simulink model "W02_Base_Map_PB_cs"  (R2019a)
settings: Solver=FixedStepDiscrete  StartTime=0.0  StopTime=inf  FixedStep=1/300  RelTol=1e-3
PreLoadFcn:
  | mbxruntime.callbacks.PreLoadFcn(bdroot);
  | check_NUTS_defined
  | model_closed = 0;
  | assignin('base',['model_closed_' bdroot],false);
PostLoadFcn:
  | mbxruntime.callbacks.PostLoadFcn(bdroot);
InitFcn:
  | mbxruntime.callbacks.InitFcn(bdroot);
StartFcn:
  | mbxruntime.callbacks.StartFcn(bdroot);
StopFcn:
  | mbxruntime.callbacks.StopFcn(bdroot);;
  | 
model workspace: external: MAT-File .\W02_Base_Map_PB_cs_hws.mat (data not in the file)
undefined symbols (not defined in the file or in its folder): DiscIntNeverNeededParam, Header, InitImageOutputDir, mbxruntime, Orientation, Pose, Poses, Poses_SL_Info, Position, tabledata
libraries: PBCSimulinkLibrary x57, simulink_extras x9, PreScanSimulinkLibrary x6, robotlib x6, PreScanUsefulBlocks x4, sharedtransform x3, aerolibutil x2, visionconversions x1, visionsinks x1
(part 3 of 7)

== system W02_Base_Map_PB_cs/TrafficLightRoadSideNL_1 ==
  note: Light SPD Resources
      |
      |  0: CIE_A_standard_incandescent_illuminant.txt
      |  1: CIE_A_standard_incandescent_illuminant.txt_x_R255_G191_B000.txt
      |  2: CIE_A_standard_incandescent_illuminant.txt_x_R583_G047_B000.txt
      |  3: CIE_F12_standard_fluorescent_illuminant.txt
      |  4: Illuminant_D65.txt
      |  5: Light_SPD_H1_12_8V_Filament.txt
      |  6: Light_SPD_H1_13_2V_Filament.txt
      |  7: Light_SPD_H11_12V_Filament.txt
      |  8: Light_SPD_H7_12_8V_Filament.txt
      |  9: Light_SPD_H7_13_2V_Filament.txt
      | 10: Light_SPD_H8_13_2V_Filament.txt
      | 11: Light_SPD_Halogen.txt
      | 12: Light_SPD_High_Power_LED.txt
      | 13: Light_SPD_HPS_High_Pressure_Sodium.txt
      | 14: Light_SPD_incandescent_traffic_signal_amber.txt
      | 15: Light_SPD_incandescent_traffic_signal_green.txt
      | 16: Light_SPD_incandescent_traffic_signal_red.txt
      | 17: Light_SPD_LED_D1S_HID.txt
      | 18: Light_SPD_LED_traffic_signal_amber.txt
      | 19: Light_SPD_LED_traffic_signal_green.txt
      | 20: Light_SPD_LED_traffic_signal_red.txt
      | 21: Light_SPD_LPS_Low_Pressure_Sodium.txt
      | 22: Light_SPD_Mercury.txt
      | 23: Light_SPD_Reddish_Neon_Sign.txt
      | 24: Noma_Twister_Blue_13W_120V.txt
      | 25: Philips_Blue_Golite_P1_Apollo_1750Lux.txt
      | 26: SPD_flat_1.0.txt
  note: Light SPD Resources
  Ground_1 : Ground
  Ground_2 : Ground
  Ground_3 : Ground
  TrafficLightRoadSideNL_1_Casing.LightGreen_Control_Mux : Subsystem  Tag=mux/plugin/LightSignals
  TrafficLightRoadSideNL_1_Casing.LightGreen_Power : Constant  Tag=TrafficLightRoadSideNL_1_Casing.LightGreen_Power  Value=0
  TrafficLightRoadSideNL_1_Casing.LightGreen_SPDIndex : Constant  Tag=TrafficLightRoadSideNL_1_Casing.LightGreen_SPDIndex  Value=15
  TrafficLightRoadSideNL_1_Casing.LightOrange_Control_Mux : Subsystem  Tag=mux/plugin/LightSignals
  TrafficLightRoadSideNL_1_Casing.LightOrange_Power : Constant  Tag=TrafficLightRoadSideNL_1_Casing.LightOrange_Power  Value=0
  TrafficLightRoadSideNL_1_Casing.LightOrange_SPDIndex : Constant  Tag=TrafficLightRoadSideNL_1_Casing.LightOrange_SPDIndex  Value=14
  TrafficLightRoadSideNL_1_Casing.LightRed_Control_Mux : Subsystem  Tag=mux/plugin/LightSignals
  TrafficLightRoadSideNL_1_Casing.LightRed_Power : Constant  Tag=TrafficLightRoadSideNL_1_Casing.LightRed_Power  Value=0
  TrafficLightRoadSideNL_1_Casing.LightRed_SPDIndex : Constant  Tag=TrafficLightRoadSideNL_1_Casing.LightRed_SPDIndex  Value=16
  VISUCasingLights_Mux : Subsystem  Tag=mux/VisuCasingLights  mask(PreScan User Interface: VisuTrafficLight){}
      mask help:
      | The VisuTrafficLight block provides a way to animate traffic lights: switch on and off individual lights.
      |
      | For more information, please click Help.
      mask Help: eval('openHelp(731)')
  VISUCasingLights_TrafficLightRoadSideNL_1 : Outport  Tag=outport/VisuCasingLights  SampleTime=1/300
  TrafficLightRoadSideNL_1_Casing.LightRed_Control : Outport  Tag=outport/plugin/sfun_PBCLight  Port=2  OutDataTypeStr=Bus: PRESCAN_PBCLIGHT_DATA  PortDimensions=1  SampleTime=0.05
  TrafficLightRoadSideNL_1_Casing.LightOrange_Control : Outport  Tag=outport/plugin/sfun_PBCLight  Port=3  OutDataTypeStr=Bus: PRESCAN_PBCLIGHT_DATA  PortDimensions=1  SampleTime=0.05
  TrafficLightRoadSideNL_1_Casing.LightGreen_Control : Outport  Tag=outport/plugin/sfun_PBCLight  Port=4  OutDataTypeStr=Bus: PRESCAN_PBCLIGHT_DATA  PortDimensions=1  SampleTime=0.05
  wires:
  VISUCasingLights_Mux/1(VISUCasingLights_TrafficLightRoadSideNL_1) -> VISUCasingLights_TrafficLightRoadSideNL_1/1
  TrafficLightRoadSideNL_1_Casing.LightRed_Control_Mux/1(Bus) -> TrafficLightRoadSideNL_1_Casing.LightRed_Control/1
  TrafficLightRoadSideNL_1_Casing.LightRed_SPDIndex/1 -> TrafficLightRoadSideNL_1_Casing.LightRed_Control_Mux/1(SPDIndex [-])
  TrafficLightRoadSideNL_1_Casing.LightRed_Power/1 -> TrafficLightRoadSideNL_1_Casing.LightRed_Control_Mux/2(Power [W])
  TrafficLightRoadSideNL_1_Casing.LightOrange_Control_Mux/1(Bus) -> TrafficLightRoadSideNL_1_Casing.LightOrange_Control/1
  TrafficLightRoadSideNL_1_Casing.LightOrange_SPDIndex/1 -> TrafficLightRoadSideNL_1_Casing.LightOrange_Control_Mux/1(SPDIndex [-])
  TrafficLightRoadSideNL_1_Casing.LightOrange_Power/1 -> TrafficLightRoadSideNL_1_Casing.LightOrange_Control_Mux/2(Power [W])
  TrafficLightRoadSideNL_1_Casing.LightGreen_Control_Mux/1(Bus) -> TrafficLightRoadSideNL_1_Casing.LightGreen_Control/1
  TrafficLightRoadSideNL_1_Casing.LightGreen_SPDIndex/1 -> TrafficLightRoadSideNL_1_Casing.LightGreen_Control_Mux/1(SPDIndex [-])
  TrafficLightRoadSideNL_1_Casing.LightGreen_Power/1 -> TrafficLightRoadSideNL_1_Casing.LightGreen_Control_Mux/2(Power [W])
  Ground_1/1 -> VISUCasingLights_Mux/1(Green [-])
  Ground_2/1 -> VISUCasingLights_Mux/2(Orange [-])
  Ground_3/1 -> VISUCasingLights_Mux/3(Red [-])

== system W02_Base_Map_PB_cs/TrafficLightRoadSideNL_1_Casing.LightGreen_Control ==
  TrafficLightRoadSideNL_1_Casing.LightGreen_Control : Inport  Tag=inport/plugin/sfun_PBCLight  OutDataTypeStr=Bus: PRESCAN_PBCLIGHT_DATA  PortDimensions=1  SampleTime=0.05  BusOutputAsStruct=on
  Actuator : S-Function  LoadFcn=addpath 'C:/Program Files/Simcenter Prescan/Prescan_2019.2/Plugins/PBCameraPlugin/matlab';addpath 'C:/Program Files/Simcenter Prescan/Prescan_2019.2/Plugins/PBCameraPlugin/bin';load('PreScanPBCLightData.mat');  FunctionName=sfun_PBCLight  Parameters=lightID, timestepMask  SFunctionDeploymentMode=off  EnableBusSupport=off  mask(Physics Based Camera plugin block){lightID=2, timestepMask=0.05}
      mask prompts: lightID "Light ID:"; timestepMask "MATLAB timestep:"
      mask help: Light Control I/O
      mask Help: eval('openHelp(6500)')
      mask Display: image(imread('ico_PBCControl.png'))
  wires:
  TrafficLightRoadSideNL_1_Casing.LightGreen_Control/1 -> Actuator/1

== system W02_Base_Map_PB_cs/TrafficLightRoadSideNL_1_Casing.LightOrange_Control ==
  TrafficLightRoadSideNL_1_Casing.LightOrange_Control : Inport  Tag=inport/plugin/sfun_PBCLight  OutDataTypeStr=Bus: PRESCAN_PBCLIGHT_DATA  PortDimensions=1  SampleTime=0.05  BusOutputAsStruct=on
  Actuator : S-Function  LoadFcn=addpath 'C:/Program Files/Simcenter Prescan/Prescan_2019.2/Plugins/PBCameraPlugin/matlab';addpath 'C:/Program Files/Simcenter Prescan/Prescan_2019.2/Plugins/PBCameraPlugin/bin';load('PreScanPBCLightData.mat');  FunctionName=sfun_PBCLight  Parameters=lightID, timestepMask  SFunctionDeploymentMode=off  EnableBusSupport=off  mask(Physics Based Camera plugin block){lightID=1, timestepMask=0.05}
      mask prompts: lightID "Light ID:"; timestepMask "MATLAB timestep:"
      mask help: Light Control I/O
      mask Help: eval('openHelp(6500)')
      mask Display: image(imread('ico_PBCControl.png'))
  wires:
  TrafficLightRoadSideNL_1_Casing.LightOrange_Control/1 -> Actuator/1

== system W02_Base_Map_PB_cs/TrafficLightRoadSideNL_1_Casing.LightRed_Control ==
  TrafficLightRoadSideNL_1_Casing.LightRed_Control : Inport  Tag=inport/plugin/sfun_PBCLight  OutDataTypeStr=Bus: PRESCAN_PBCLIGHT_DATA  PortDimensions=1  SampleTime=0.05  BusOutputAsStruct=on
  Actuator : S-Function  LoadFcn=addpath 'C:/Program Files/Simcenter Prescan/Prescan_2019.2/Plugins/PBCameraPlugin/matlab';addpath 'C:/Program Files/Simcenter Prescan/Prescan_2019.2/Plugins/PBCameraPlugin/bin';load('PreScanPBCLightData.mat');  FunctionName=sfun_PBCLight  Parameters=lightID, timestepMask  SFunctionDeploymentMode=off  EnableBusSupport=off  mask(Physics Based Camera plugin block){lightID=0, timestepMask=0.05}
      mask prompts: lightID "Light ID:"; timestepMask "MATLAB timestep:"
      mask help: Light Control I/O
      mask Help: eval('openHelp(6500)')
      mask Display: image(imread('ico_PBCControl.png'))
  wires:
  TrafficLightRoadSideNL_1_Casing.LightRed_Control/1 -> Actuator/1

== system W02_Base_Map_PB_cs/TrafficLightRoadSideNL_2 ==
  note: Light SPD Resources
      |
      |  0: CIE_A_standard_incandescent_illuminant.txt
      |  1: CIE_A_standard_incandescent_illuminant.txt_x_R255_G191_B000.txt
      |  2: CIE_A_standard_incandescent_illuminant.txt_x_R583_G047_B000.txt
      |  3: CIE_F12_standard_fluorescent_illuminant.txt
      |  4: Illuminant_D65.txt
      |  5: Light_SPD_H1_12_8V_Filament.txt
      |  6: Light_SPD_H1_13_2V_Filament.txt
      |  7: Light_SPD_H11_12V_Filament.txt
      |  8: Light_SPD_H7_12_8V_Filament.txt
      |  9: Light_SPD_H7_13_2V_Filament.txt
      | 10: Light_SPD_H8_13_2V_Filament.txt
      | 11: Light_SPD_Halogen.txt
      | 12: Light_SPD_High_Power_LED.txt
      | 13: Light_SPD_HPS_High_Pressure_Sodium.txt
      | 14: Light_SPD_incandescent_traffic_signal_amber.txt
      | 15: Light_SPD_incandescent_traffic_signal_green.txt
      | 16: Light_SPD_incandescent_traffic_signal_red.txt
      | 17: Light_SPD_LED_D1S_HID.txt
      | 18: Light_SPD_LED_traffic_signal_amber.txt
      | 19: Light_SPD_LED_traffic_signal_green.txt
      | 20: Light_SPD_LED_traffic_signal_red.txt
      | 21: Light_SPD_LPS_Low_Pressure_Sodium.txt
      | 22: Light_SPD_Mercury.txt
      | 23: Light_SPD_Reddish_Neon_Sign.txt
      | 24: Noma_Twister_Blue_13W_120V.txt
      | 25: Philips_Blue_Golite_P1_Apollo_1750Lux.txt
      | 26: SPD_flat_1.0.txt
  note: Light SPD Resources
  Ground_1 : Ground
  Ground_2 : Ground
  Ground_3 : Ground
  TrafficLightRoadSideNL_2_Casing.LightGreen_Control_Mux : Subsystem  Tag=mux/plugin/LightSignals
  TrafficLightRoadSideNL_2_Casing.LightGreen_Power : Constant  Tag=TrafficLightRoadSideNL_2_Casing.LightGreen_Power  Value=0
  TrafficLightRoadSideNL_2_Casing.LightGreen_SPDIndex : Constant  Tag=TrafficLightRoadSideNL_2_Casing.LightGreen_SPDIndex  Value=15
  TrafficLightRoadSideNL_2_Casing.LightOrange_Control_Mux : Subsystem  Tag=mux/plugin/LightSignals
  TrafficLightRoadSideNL_2_Casing.LightOrange_Power : Constant  Tag=TrafficLightRoadSideNL_2_Casing.LightOrange_Power  Value=0
  TrafficLightRoadSideNL_2_Casing.LightOrange_SPDIndex : Constant  Tag=TrafficLightRoadSideNL_2_Casing.LightOrange_SPDIndex  Value=14
  TrafficLightRoadSideNL_2_Casing.LightRed_Control_Mux : Subsystem  Tag=mux/plugin/LightSignals
  TrafficLightRoadSideNL_2_Casing.LightRed_Power : Constant  Tag=TrafficLightRoadSideNL_2_Casing.LightRed_Power  Value=0
  TrafficLightRoadSideNL_2_Casing.LightRed_SPDIndex : Constant  Tag=TrafficLightRoadSideNL_2_Casing.LightRed_SPDIndex  Value=16
  VISUCasingLights_Mux : Subsystem  Tag=mux/VisuCasingLights  mask(PreScan User Interface: VisuTrafficLight){}
      mask help:
      | The VisuTrafficLight block provides a way to animate traffic lights: switch on and off individual lights.
      |
      | For more information, please click Help.
      mask Help: eval('openHelp(731)')
  VISUCasingLights_TrafficLightRoadSideNL_2 : Outport  Tag=outport/VisuCasingLights  SampleTime=1/300
  TrafficLightRoadSideNL_2_Casing.LightRed_Control : Outport  Tag=outport/plugin/sfun_PBCLight  Port=2  OutDataTypeStr=Bus: PRESCAN_PBCLIGHT_DATA  PortDimensions=1  SampleTime=0.05
  TrafficLightRoadSideNL_2_Casing.LightOrange_Control : Outport  Tag=outport/plugin/sfun_PBCLight  Port=3  OutDataTypeStr=Bus: PRESCAN_PBCLIGHT_DATA  PortDimensions=1  SampleTime=0.05
  TrafficLightRoadSideNL_2_Casing.LightGreen_Control : Outport  Tag=outport/plugin/sfun_PBCLight  Port=4  OutDataTypeStr=Bus: PRESCAN_PBCLIGHT_DATA  PortDimensions=1  SampleTime=0.05
  wires:
  VISUCasingLights_Mux/1(VISUCasingLights_TrafficLightRoadSideNL_2) -> VISUCasingLights_TrafficLightRoadSideNL_2/1
  TrafficLightRoadSideNL_2_Casing.LightRed_Control_Mux/1(Bus) -> TrafficLightRoadSideNL_2_Casing.LightRed_Control/1
  TrafficLightRoadSideNL_2_Casing.LightRed_SPDIndex/1 -> TrafficLightRoadSideNL_2_Casing.LightRed_Control_Mux/1(SPDIndex [-])
  TrafficLightRoadSideNL_2_Casing.LightRed_Power/1 -> TrafficLightRoadSideNL_2_Casing.LightRed_Control_Mux/2(Power [W])
  TrafficLightRoadSideNL_2_Casing.LightOrange_Control_Mux/1(Bus) -> TrafficLightRoadSideNL_2_Casing.LightOrange_Control/1
  TrafficLightRoadSideNL_2_Casing.LightOrange_SPDIndex/1 -> TrafficLightRoadSideNL_2_Casing.LightOrange_Control_Mux/1(SPDIndex [-])
  TrafficLightRoadSideNL_2_Casing.LightOrange_Power/1 -> TrafficLightRoadSideNL_2_Casing.LightOrange_Control_Mux/2(Power [W])
  TrafficLightRoadSideNL_2_Casing.LightGreen_Control_Mux/1(Bus) -> TrafficLightRoadSideNL_2_Casing.LightGreen_Control/1
  TrafficLightRoadSideNL_2_Casing.LightGreen_SPDIndex/1 -> TrafficLightRoadSideNL_2_Casing.LightGreen_Control_Mux/1(SPDIndex [-])
  TrafficLightRoadSideNL_2_Casing.LightGreen_Power/1 -> TrafficLightRoadSideNL_2_Casing.LightGreen_Control_Mux/2(Power [W])
  Ground_1/1 -> VISUCasingLights_Mux/1(Green [-])
  Ground_2/1 -> VISUCasingLights_Mux/2(Orange [-])
  Ground_3/1 -> VISUCasingLights_Mux/3(Red [-])

== system W02_Base_Map_PB_cs/TrafficLightRoadSideNL_2_Casing.LightGreen_Control ==
  TrafficLightRoadSideNL_2_Casing.LightGreen_Control : Inport  Tag=inport/plugin/sfun_PBCLight  OutDataTypeStr=Bus: PRESCAN_PBCLIGHT_DATA  PortDimensions=1  SampleTime=0.05  BusOutputAsStruct=on
  Actuator : S-Function  LoadFcn=addpath 'C:/Program Files/Simcenter Prescan/Prescan_2019.2/Plugins/PBCameraPlugin/matlab';addpath 'C:/Program Files/Simcenter Prescan/Prescan_2019.2/Plugins/PBCameraPlugin/bin';load('PreScanPBCLightData.mat');  FunctionName=sfun_PBCLight  Parameters=lightID, timestepMask  SFunctionDeploymentMode=off  EnableBusSupport=off  mask(Physics Based Camera plugin block){lightID=5, timestepMask=0.05}
      mask prompts: lightID "Light ID:"; timestepMask "MATLAB timestep:"
      mask help: Light Control I/O
      mask Help: eval('openHelp(6500)')
      mask Display: image(imread('ico_PBCControl.png'))
  wires:
  TrafficLightRoadSideNL_2_Casing.LightGreen_Control/1 -> Actuator/1

== system W02_Base_Map_PB_cs/TrafficLightRoadSideNL_2_Casing.LightOrange_Control ==
  TrafficLightRoadSideNL_2_Casing.LightOrange_Control : Inport  Tag=inport/plugin/sfun_PBCLight  OutDataTypeStr=Bus: PRESCAN_PBCLIGHT_DATA  PortDimensions=1  SampleTime=0.05  BusOutputAsStruct=on
  Actuator : S-Function  LoadFcn=addpath 'C:/Program Files/Simcenter Prescan/Prescan_2019.2/Plugins/PBCameraPlugin/matlab';addpath 'C:/Program Files/Simcenter Prescan/Prescan_2019.2/Plugins/PBCameraPlugin/bin';load('PreScanPBCLightData.mat');  FunctionName=sfun_PBCLight  Parameters=lightID, timestepMask  SFunctionDeploymentMode=off  EnableBusSupport=off  mask(Physics Based Camera plugin block){lightID=4, timestepMask=0.05}
      mask prompts: lightID "Light ID:"; timestepMask "MATLAB timestep:"
      mask help: Light Control I/O
      mask Help: eval('openHelp(6500)')
      mask Display: image(imread('ico_PBCControl.png'))
  wires:
  TrafficLightRoadSideNL_2_Casing.LightOrange_Control/1 -> Actuator/1

== system W02_Base_Map_PB_cs/TrafficLightRoadSideNL_2_Casing.LightRed_Control ==
  TrafficLightRoadSideNL_2_Casing.LightRed_Control : Inport  Tag=inport/plugin/sfun_PBCLight  OutDataTypeStr=Bus: PRESCAN_PBCLIGHT_DATA  PortDimensions=1  SampleTime=0.05  BusOutputAsStruct=on
  Actuator : S-Function  LoadFcn=addpath 'C:/Program Files/Simcenter Prescan/Prescan_2019.2/Plugins/PBCameraPlugin/matlab';addpath 'C:/Program Files/Simcenter Prescan/Prescan_2019.2/Plugins/PBCameraPlugin/bin';load('PreScanPBCLightData.mat');  FunctionName=sfun_PBCLight  Parameters=lightID, timestepMask  SFunctionDeploymentMode=off  EnableBusSupport=off  mask(Physics Based Camera plugin block){lightID=3, timestepMask=0.05}
      mask prompts: lightID "Light ID:"; timestepMask "MATLAB timestep:"
      mask help: Light Control I/O
      mask Help: eval('openHelp(6500)')
      mask Display: image(imread('ico_PBCControl.png'))
  wires:
  TrafficLightRoadSideNL_2_Casing.LightRed_Control/1 -> Actuator/1

== system W02_Base_Map_PB_cs/TrafficLightRoadSideNL_3 ==
  note: Light SPD Resources
      |
      |  0: CIE_A_standard_incandescent_illuminant.txt
      |  1: CIE_A_standard_incandescent_illuminant.txt_x_R255_G191_B000.txt
      |  2: CIE_A_standard_incandescent_illuminant.txt_x_R583_G047_B000.txt
      |  3: CIE_F12_standard_fluorescent_illuminant.txt
      |  4: Illuminant_D65.txt
      |  5: Light_SPD_H1_12_8V_Filament.txt
      |  6: Light_SPD_H1_13_2V_Filament.txt
      |  7: Light_SPD_H11_12V_Filament.txt
      |  8: Light_SPD_H7_12_8V_Filament.txt
      |  9: Light_SPD_H7_13_2V_Filament.txt
      | 10: Light_SPD_H8_13_2V_Filament.txt
      | 11: Light_SPD_Halogen.txt
      | 12: Light_SPD_High_Power_LED.txt
      | 13: Light_SPD_HPS_High_Pressure_Sodium.txt
      | 14: Light_SPD_incandescent_traffic_signal_amber.txt
      | 15: Light_SPD_incandescent_traffic_signal_green.txt
      | 16: Light_SPD_incandescent_traffic_signal_red.txt
      | 17: Light_SPD_LED_D1S_HID.txt
      | 18: Light_SPD_LED_traffic_signal_amber.txt
      | 19: Light_SPD_LED_traffic_signal_green.txt
      | 20: Light_SPD_LED_traffic_signal_red.txt
      | 21: Light_SPD_LPS_Low_Pressure_Sodium.txt
      | 22: Light_SPD_Mercury.txt
      | 23: Light_SPD_Reddish_Neon_Sign.txt
      | 24: Noma_Twister_Blue_13W_120V.txt
      | 25: Philips_Blue_Golite_P1_Apollo_1750Lux.txt
      | 26: SPD_flat_1.0.txt
  note: Light SPD Resources
  Ground_1 : Ground
  Ground_2 : Ground
  Ground_3 : Ground
  TrafficLightRoadSideNL_3_Casing.LightGreen_Control_Mux : Subsystem  Tag=mux/plugin/LightSignals
  TrafficLightRoadSideNL_3_Casing.LightGreen_Power : Constant  Tag=TrafficLightRoadSideNL_3_Casing.LightGreen_Power  Value=0
  TrafficLightRoadSideNL_3_Casing.LightGreen_SPDIndex : Constant  Tag=TrafficLightRoadSideNL_3_Casing.LightGreen_SPDIndex  Value=15
  TrafficLightRoadSideNL_3_Casing.LightOrange_Control_Mux : Subsystem  Tag=mux/plugin/LightSignals
  TrafficLightRoadSideNL_3_Casing.LightOrange_Power : Constant  Tag=TrafficLightRoadSideNL_3_Casing.LightOrange_Power  Value=0
  TrafficLightRoadSideNL_3_Casing.LightOrange_SPDIndex : Constant  Tag=TrafficLightRoadSideNL_3_Casing.LightOrange_SPDIndex  Value=14
  TrafficLightRoadSideNL_3_Casing.LightRed_Control_Mux : Subsystem  Tag=mux/plugin/LightSignals
  TrafficLightRoadSideNL_3_Casing.LightRed_Power : Constant  Tag=TrafficLightRoadSideNL_3_Casing.LightRed_Power  Value=0
  TrafficLightRoadSideNL_3_Casing.LightRed_SPDIndex : Constant  Tag=TrafficLightRoadSideNL_3_Casing.LightRed_SPDIndex  Value=16
  VISUCasingLights_Mux : Subsystem  Tag=mux/VisuCasingLights  mask(PreScan User Interface: VisuTrafficLight){}
      mask help:
      | The VisuTrafficLight block provides a way to animate traffic lights: switch on and off individual lights.
      |
      | For more information, please click Help.
      mask Help: eval('openHelp(731)')
  VISUCasingLights_TrafficLightRoadSideNL_3 : Outport  Tag=outport/VisuCasingLights  SampleTime=1/300
  TrafficLightRoadSideNL_3_Casing.LightRed_Control : Outport  Tag=outport/plugin/sfun_PBCLight  Port=2  OutDataTypeStr=Bus: PRESCAN_PBCLIGHT_DATA  PortDimensions=1  SampleTime=0.05
  TrafficLightRoadSideNL_3_Casing.LightOrange_Control : Outport  Tag=outport/plugin/sfun_PBCLight  Port=3  OutDataTypeStr=Bus: PRESCAN_PBCLIGHT_DATA  PortDimensions=1  SampleTime=0.05
  TrafficLightRoadSideNL_3_Casing.LightGreen_Control : Outport  Tag=outport/plugin/sfun_PBCLight  Port=4  OutDataTypeStr=Bus: PRESCAN_PBCLIGHT_DATA  PortDimensions=1  SampleTime=0.05
  wires:
  VISUCasingLights_Mux/1(VISUCasingLights_TrafficLightRoadSideNL_3) -> VISUCasingLights_TrafficLightRoadSideNL_3/1
  TrafficLightRoadSideNL_3_Casing.LightRed_Control_Mux/1(Bus) -> TrafficLightRoadSideNL_3_Casing.LightRed_Control/1
  TrafficLightRoadSideNL_3_Casing.LightRed_SPDIndex/1 -> TrafficLightRoadSideNL_3_Casing.LightRed_Control_Mux/1(SPDIndex [-])
  TrafficLightRoadSideNL_3_Casing.LightRed_Power/1 -> TrafficLightRoadSideNL_3_Casing.LightRed_Control_Mux/2(Power [W])
  TrafficLightRoadSideNL_3_Casing.LightOrange_Control_Mux/1(Bus) -> TrafficLightRoadSideNL_3_Casing.LightOrange_Control/1
  TrafficLightRoadSideNL_3_Casing.LightOrange_SPDIndex/1 -> TrafficLightRoadSideNL_3_Casing.LightOrange_Control_Mux/1(SPDIndex [-])
  TrafficLightRoadSideNL_3_Casing.LightOrange_Power/1 -> TrafficLightRoadSideNL_3_Casing.LightOrange_Control_Mux/2(Power [W])
  TrafficLightRoadSideNL_3_Casing.LightGreen_Control_Mux/1(Bus) -> TrafficLightRoadSideNL_3_Casing.LightGreen_Control/1
  TrafficLightRoadSideNL_3_Casing.LightGreen_SPDIndex/1 -> TrafficLightRoadSideNL_3_Casing.LightGreen_Control_Mux/1(SPDIndex [-])
  TrafficLightRoadSideNL_3_Casing.LightGreen_Power/1 -> TrafficLightRoadSideNL_3_Casing.LightGreen_Control_Mux/2(Power [W])
  Ground_1/1 -> VISUCasingLights_Mux/1(Green [-])
  Ground_2/1 -> VISUCasingLights_Mux/2(Orange [-])
  Ground_3/1 -> VISUCasingLights_Mux/3(Red [-])

== system W02_Base_Map_PB_cs/TrafficLightRoadSideNL_3_Casing.LightGreen_Control ==
  TrafficLightRoadSideNL_3_Casing.LightGreen_Control : Inport  Tag=inport/plugin/sfun_PBCLight  OutDataTypeStr=Bus: PRESCAN_PBCLIGHT_DATA  PortDimensions=1  SampleTime=0.05  BusOutputAsStruct=on
  Actuator : S-Function  LoadFcn=addpath 'C:/Program Files/Simcenter Prescan/Prescan_2019.2/Plugins/PBCameraPlugin/matlab';addpath 'C:/Program Files/Simcenter Prescan/Prescan_2019.2/Plugins/PBCameraPlugin/bin';load('PreScanPBCLightData.mat');  FunctionName=sfun_PBCLight  Parameters=lightID, timestepMask  SFunctionDeploymentMode=off  EnableBusSupport=off  mask(Physics Based Camera plugin block){lightID=8, timestepMask=0.05}
      mask prompts: lightID "Light ID:"; timestepMask "MATLAB timestep:"
      mask help: Light Control I/O
      mask Help: eval('openHelp(6500)')
      mask Display: image(imread('ico_PBCControl.png'))
  wires:
  TrafficLightRoadSideNL_3_Casing.LightGreen_Control/1 -> Actuator/1

== system W02_Base_Map_PB_cs/TrafficLightRoadSideNL_3_Casing.LightOrange_Control ==
  TrafficLightRoadSideNL_3_Casing.LightOrange_Control : Inport  Tag=inport/plugin/sfun_PBCLight  OutDataTypeStr=Bus: PRESCAN_PBCLIGHT_DATA  PortDimensions=1  SampleTime=0.05  BusOutputAsStruct=on
  Actuator : S-Function  LoadFcn=addpath 'C:/Program Files/Simcenter Prescan/Prescan_2019.2/Plugins/PBCameraPlugin/matlab';addpath 'C:/Program Files/Simcenter Prescan/Prescan_2019.2/Plugins/PBCameraPlugin/bin';load('PreScanPBCLightData.mat');  FunctionName=sfun_PBCLight  Parameters=lightID, timestepMask  SFunctionDeploymentMode=off  EnableBusSupport=off  mask(Physics Based Camera plugin block){lightID=7, timestepMask=0.05}
      mask prompts: lightID "Light ID:"; timestepMask "MATLAB timestep:"
      mask help: Light Control I/O
      mask Help: eval('openHelp(6500)')
      mask Display: image(imread('ico_PBCControl.png'))
  wires:
  TrafficLightRoadSideNL_3_Casing.LightOrange_Control/1 -> Actuator/1

== system W02_Base_Map_PB_cs/TrafficLightRoadSideNL_3_Casing.LightRed_Control ==
  TrafficLightRoadSideNL_3_Casing.LightRed_Control : Inport  Tag=inport/plugin/sfun_PBCLight  OutDataTypeStr=Bus: PRESCAN_PBCLIGHT_DATA  PortDimensions=1  SampleTime=0.05  BusOutputAsStruct=on
  Actuator : S-Function  LoadFcn=addpath 'C:/Program Files/Simcenter Prescan/Prescan_2019.2/Plugins/PBCameraPlugin/matlab';addpath 'C:/Program Files/Simcenter Prescan/Prescan_2019.2/Plugins/PBCameraPlugin/bin';load('PreScanPBCLightData.mat');  FunctionName=sfun_PBCLight  Parameters=lightID, timestepMask  SFunctionDeploymentMode=off  EnableBusSupport=off  mask(Physics Based Camera plugin block){lightID=6, timestepMask=0.05}
      mask prompts: lightID "Light ID:"; timestepMask "MATLAB timestep:"
      mask help: Light Control I/O
      mask Help: eval('openHelp(6500)')
      mask Display: image(imread('ico_PBCControl.png'))
  wires:
  TrafficLightRoadSideNL_3_Casing.LightRed_Control/1 -> Actuator/1

== system W02_Base_Map_PB_cs/TrafficLightRoadSideNL_4 ==
  note: Light SPD Resources
      |
      |  0: CIE_A_standard_incandescent_illuminant.txt
      |  1: CIE_A_standard_incandescent_illuminant.txt_x_R255_G191_B000.txt
      |  2: CIE_A_standard_incandescent_illuminant.txt_x_R583_G047_B000.txt
      |  3: CIE_F12_standard_fluorescent_illuminant.txt
      |  4: Illuminant_D65.txt
      |  5: Light_SPD_H1_12_8V_Filament.txt
      |  6: Light_SPD_H1_13_2V_Filament.txt
      |  7: Light_SPD_H11_12V_Filament.txt
      |  8: Light_SPD_H7_12_8V_Filament.txt
      |  9: Light_SPD_H7_13_2V_Filament.txt
      | 10: Light_SPD_H8_13_2V_Filament.txt
      | 11: Light_SPD_Halogen.txt
      | 12: Light_SPD_High_Power_LED.txt
      | 13: Light_SPD_HPS_High_Pressure_Sodium.txt
      | 14: Light_SPD_incandescent_traffic_signal_amber.txt
      | 15: Light_SPD_incandescent_traffic_signal_green.txt
      | 16: Light_SPD_incandescent_traffic_signal_red.txt
      | 17: Light_SPD_LED_D1S_HID.txt
      | 18: Light_SPD_LED_traffic_signal_amber.txt
      | 19: Light_SPD_LED_traffic_signal_green.txt
      | 20: Light_SPD_LED_traffic_signal_red.txt
      | 21: Light_SPD_LPS_Low_Pressure_Sodium.txt
      | 22: Light_SPD_Mercury.txt
      | 23: Light_SPD_Reddish_Neon_Sign.txt
      | 24: Noma_Twister_Blue_13W_120V.txt
      | 25: Philips_Blue_Golite_P1_Apollo_1750Lux.txt
      | 26: SPD_flat_1.0.txt
  note: Light SPD Resources
  Ground_1 : Ground
  Ground_2 : Ground
  Ground_3 : Ground
  TrafficLightRoadSideNL_4_Casing.LightGreen_Control_Mux : Subsystem  Tag=mux/plugin/LightSignals
  TrafficLightRoadSideNL_4_Casing.LightGreen_Power : Constant  Tag=TrafficLightRoadSideNL_4_Casing.LightGreen_Power  Value=0
  TrafficLightRoadSideNL_4_Casing.LightGreen_SPDIndex : Constant  Tag=TrafficLightRoadSideNL_4_Casing.LightGreen_SPDIndex  Value=15
  TrafficLightRoadSideNL_4_Casing.LightOrange_Control_Mux : Subsystem  Tag=mux/plugin/LightSignals
  TrafficLightRoadSideNL_4_Casing.LightOrange_Power : Constant  Tag=TrafficLightRoadSideNL_4_Casing.LightOrange_Power  Value=0
  TrafficLightRoadSideNL_4_Casing.LightOrange_SPDIndex : Constant  Tag=TrafficLightRoadSideNL_4_Casing.LightOrange_SPDIndex  Value=14
  TrafficLightRoadSideNL_4_Casing.LightRed_Control_Mux : Subsystem  Tag=mux/plugin/LightSignals
  TrafficLightRoadSideNL_4_Casing.LightRed_Power : Constant  Tag=TrafficLightRoadSideNL_4_Casing.LightRed_Power  Value=0
  TrafficLightRoadSideNL_4_Casing.LightRed_SPDIndex : Constant  Tag=TrafficLightRoadSideNL_4_Casing.LightRed_SPDIndex  Value=16
  VISUCasingLights_Mux : Subsystem  Tag=mux/VisuCasingLights  mask(PreScan User Interface: VisuTrafficLight){}
      mask help:
      | The VisuTrafficLight block provides a way to animate traffic lights: switch on and off individual lights.
      |
      | For more information, please click Help.
      mask Help: eval('openHelp(731)')
  VISUCasingLights_TrafficLightRoadSideNL_4 : Outport  Tag=outport/VisuCasingLights  SampleTime=1/300
  TrafficLightRoadSideNL_4_Casing.LightRed_Control : Outport  Tag=outport/plugin/sfun_PBCLight  Port=2  OutDataTypeStr=Bus: PRESCAN_PBCLIGHT_DATA  PortDimensions=1  SampleTime=0.05
  TrafficLightRoadSideNL_4_Casing.LightOrange_Control : Outport  Tag=outport/plugin/sfun_PBCLight  Port=3  OutDataTypeStr=Bus: PRESCAN_PBCLIGHT_DATA  PortDimensions=1  SampleTime=0.05
  TrafficLightRoadSideNL_4_Casing.LightGreen_Control : Outport  Tag=outport/plugin/sfun_PBCLight  Port=4  OutDataTypeStr=Bus: PRESCAN_PBCLIGHT_DATA  PortDimensions=1  SampleTime=0.05
  wires:
  VISUCasingLights_Mux/1(VISUCasingLights_TrafficLightRoadSideNL_4) -> VISUCasingLights_TrafficLightRoadSideNL_4/1
  TrafficLightRoadSideNL_4_Casing.LightRed_Control_Mux/1(Bus) -> TrafficLightRoadSideNL_4_Casing.LightRed_Control/1
  TrafficLightRoadSideNL_4_Casing.LightRed_SPDIndex/1 -> TrafficLightRoadSideNL_4_Casing.LightRed_Control_Mux/1(SPDIndex [-])
  TrafficLightRoadSideNL_4_Casing.LightRed_Power/1 -> TrafficLightRoadSideNL_4_Casing.LightRed_Control_Mux/2(Power [W])
  TrafficLightRoadSideNL_4_Casing.LightOrange_Control_Mux/1(Bus) -> TrafficLightRoadSideNL_4_Casing.LightOrange_Control/1
  TrafficLightRoadSideNL_4_Casing.LightOrange_SPDIndex/1 -> TrafficLightRoadSideNL_4_Casing.LightOrange_Control_Mux/1(SPDIndex [-])
  TrafficLightRoadSideNL_4_Casing.LightOrange_Power/1 -> TrafficLightRoadSideNL_4_Casing.LightOrange_Control_Mux/2(Power [W])
  TrafficLightRoadSideNL_4_Casing.LightGreen_Control_Mux/1(Bus) -> TrafficLightRoadSideNL_4_Casing.LightGreen_Control/1
  TrafficLightRoadSideNL_4_Casing.LightGreen_SPDIndex/1 -> TrafficLightRoadSideNL_4_Casing.LightGreen_Control_Mux/1(SPDIndex [-])
  TrafficLightRoadSideNL_4_Casing.LightGreen_Power/1 -> TrafficLightRoadSideNL_4_Casing.LightGreen_Control_Mux/2(Power [W])
  Ground_1/1 -> VISUCasingLights_Mux/1(Green [-])
  Ground_2/1 -> VISUCasingLights_Mux/2(Orange [-])
  Ground_3/1 -> VISUCasingLights_Mux/3(Red [-])

== system W02_Base_Map_PB_cs/TrafficLightRoadSideNL_4_Casing.LightGreen_Control ==
  TrafficLightRoadSideNL_4_Casing.LightGreen_Control : Inport  Tag=inport/plugin/sfun_PBCLight  OutDataTypeStr=Bus: PRESCAN_PBCLIGHT_DATA  PortDimensions=1  SampleTime=0.05  BusOutputAsStruct=on
  Actuator : S-Function  LoadFcn=addpath 'C:/Program Files/Simcenter Prescan/Prescan_2019.2/Plugins/PBCameraPlugin/matlab';addpath 'C:/Program Files/Simcenter Prescan/Prescan_2019.2/Plugins/PBCameraPlugin/bin';load('PreScanPBCLightData.mat');  FunctionName=sfun_PBCLight  Parameters=lightID, timestepMask  SFunctionDeploymentMode=off  EnableBusSupport=off  mask(Physics Based Camera plugin block){lightID=11, timestepMask=0.05}
      mask prompts: lightID "Light ID:"; timestepMask "MATLAB timestep:"
      mask help: Light Control I/O
      mask Help: eval('openHelp(6500)')
      mask Display: image(imread('ico_PBCControl.png'))
  wires:
  TrafficLightRoadSideNL_4_Casing.LightGreen_Control/1 -> Actuator/1

== system W02_Base_Map_PB_cs/TrafficLightRoadSideNL_4_Casing.LightOrange_Control ==
  TrafficLightRoadSideNL_4_Casing.LightOrange_Control : Inport  Tag=inport/plugin/sfun_PBCLight  OutDataTypeStr=Bus: PRESCAN_PBCLIGHT_DATA  PortDimensions=1  SampleTime=0.05  BusOutputAsStruct=on
  Actuator : S-Function  LoadFcn=addpath 'C:/Program Files/Simcenter Prescan/Prescan_2019.2/Plugins/PBCameraPlugin/matlab';addpath 'C:/Program Files/Simcenter Prescan/Prescan_2019.2/Plugins/PBCameraPlugin/bin';load('PreScanPBCLightData.mat');  FunctionName=sfun_PBCLight  Parameters=lightID, timestepMask  SFunctionDeploymentMode=off  EnableBusSupport=off  mask(Physics Based Camera plugin block){lightID=10, timestepMask=0.05}
      mask prompts: lightID "Light ID:"; timestepMask "MATLAB timestep:"
      mask help: Light Control I/O
      mask Help: eval('openHelp(6500)')
      mask Display: image(imread('ico_PBCControl.png'))
  wires:
  TrafficLightRoadSideNL_4_Casing.LightOrange_Control/1 -> Actuator/1

== system W02_Base_Map_PB_cs/TrafficLightRoadSideNL_4_Casing.LightRed_Control ==
  TrafficLightRoadSideNL_4_Casing.LightRed_Control : Inport  Tag=inport/plugin/sfun_PBCLight  OutDataTypeStr=Bus: PRESCAN_PBCLIGHT_DATA  PortDimensions=1  SampleTime=0.05  BusOutputAsStruct=on
  Actuator : S-Function  LoadFcn=addpath 'C:/Program Files/Simcenter Prescan/Prescan_2019.2/Plugins/PBCameraPlugin/matlab';addpath 'C:/Program Files/Simcenter Prescan/Prescan_2019.2/Plugins/PBCameraPlugin/bin';load('PreScanPBCLightData.mat');  FunctionName=sfun_PBCLight  Parameters=lightID, timestepMask  SFunctionDeploymentMode=off  EnableBusSupport=off  mask(Physics Based Camera plugin block){lightID=9, timestepMask=0.05}
      mask prompts: lightID "Light ID:"; timestepMask "MATLAB timestep:"
      mask help: Light Control I/O
      mask Help: eval('openHelp(6500)')
      mask Display: image(imread('ico_PBCControl.png'))
  wires:
  TrafficLightRoadSideNL_4_Casing.LightRed_Control/1 -> Actuator/1

== system W02_Base_Map_PB_cs/TrafficLightRoadSideNL_5 ==
  note: Light SPD Resources
      |
      |  0: CIE_A_standard_incandescent_illuminant.txt
      |  1: CIE_A_standard_incandescent_illuminant.txt_x_R255_G191_B000.txt
      |  2: CIE_A_standard_incandescent_illuminant.txt_x_R583_G047_B000.txt
      |  3: CIE_F12_standard_fluorescent_illuminant.txt
      |  4: Illuminant_D65.txt
      |  5: Light_SPD_H1_12_8V_Filament.txt
      |  6: Light_SPD_H1_13_2V_Filament.txt
      |  7: Light_SPD_H11_12V_Filament.txt
      |  8: Light_SPD_H7_12_8V_Filament.txt
      |  9: Light_SPD_H7_13_2V_Filament.txt
      | 10: Light_SPD_H8_13_2V_Filament.txt
      | 11: Light_SPD_Halogen.txt
      | 12: Light_SPD_High_Power_LED.txt
      | 13: Light_SPD_HPS_High_Pressure_Sodium.txt
      | 14: Light_SPD_incandescent_traffic_signal_amber.txt
      | 15: Light_SPD_incandescent_traffic_signal_green.txt
      | 16: Light_SPD_incandescent_traffic_signal_red.txt
      | 17: Light_SPD_LED_D1S_HID.txt
      | 18: Light_SPD_LED_traffic_signal_amber.txt
      | 19: Light_SPD_LED_traffic_signal_green.txt
      | 20: Light_SPD_LED_traffic_signal_red.txt
      | 21: Light_SPD_LPS_Low_Pressure_Sodium.txt
      | 22: Light_SPD_Mercury.txt
      | 23: Light_SPD_Reddish_Neon_Sign.txt
      | 24: Noma_Twister_Blue_13W_120V.txt
      | 25: Philips_Blue_Golite_P1_Apollo_1750Lux.txt
      | 26: SPD_flat_1.0.txt
  note: Light SPD Resources
  Ground_1 : Ground
  Ground_2 : Ground
  Ground_3 : Ground
  TrafficLightRoadSideNL_5_Casing.LightGreen_Control_Mux : Subsystem  Tag=mux/plugin/LightSignals
  TrafficLightRoadSideNL_5_Casing.LightGreen_Power : Constant  Tag=TrafficLightRoadSideNL_5_Casing.LightGreen_Power  Value=0
  TrafficLightRoadSideNL_5_Casing.LightGreen_SPDIndex : Constant  Tag=TrafficLightRoadSideNL_5_Casing.LightGreen_SPDIndex  Value=15
  TrafficLightRoadSideNL_5_Casing.LightOrange_Control_Mux : Subsystem  Tag=mux/plugin/LightSignals
  TrafficLightRoadSideNL_5_Casing.LightOrange_Power : Constant  Tag=TrafficLightRoadSideNL_5_Casing.LightOrange_Power  Value=0
  TrafficLightRoadSideNL_5_Casing.LightOrange_SPDIndex : Constant  Tag=TrafficLightRoadSideNL_5_Casing.LightOrange_SPDIndex  Value=14
  TrafficLightRoadSideNL_5_Casing.LightRed_Control_Mux : Subsystem  Tag=mux/plugin/LightSignals
  TrafficLightRoadSideNL_5_Casing.LightRed_Power : Constant  Tag=TrafficLightRoadSideNL_5_Casing.LightRed_Power  Value=0
  TrafficLightRoadSideNL_5_Casing.LightRed_SPDIndex : Constant  Tag=TrafficLightRoadSideNL_5_Casing.LightRed_SPDIndex  Value=16
  VISUCasingLights_Mux : Subsystem  Tag=mux/VisuCasingLights  mask(PreScan User Interface: VisuTrafficLight){}
      mask help:
      | The VisuTrafficLight block provides a way to animate traffic lights: switch on and off individual lights.
      |
      | For more information, please click Help.
      mask Help: eval('openHelp(731)')
  VISUCasingLights_TrafficLightRoadSideNL_5 : Outport  Tag=outport/VisuCasingLights  SampleTime=1/300
  TrafficLightRoadSideNL_5_Casing.LightRed_Control : Outport  Tag=outport/plugin/sfun_PBCLight  Port=2  OutDataTypeStr=Bus: PRESCAN_PBCLIGHT_DATA  PortDimensions=1  SampleTime=0.05
  TrafficLightRoadSideNL_5_Casing.LightOrange_Control : Outport  Tag=outport/plugin/sfun_PBCLight  Port=3  OutDataTypeStr=Bus: PRESCAN_PBCLIGHT_DATA  PortDimensions=1  SampleTime=0.05
  TrafficLightRoadSideNL_5_Casing.LightGreen_Control : Outport  Tag=outport/plugin/sfun_PBCLight  Port=4  OutDataTypeStr=Bus: PRESCAN_PBCLIGHT_DATA  PortDimensions=1  SampleTime=0.05
  wires:
  VISUCasingLights_Mux/1(VISUCasingLights_TrafficLightRoadSideNL_5) -> VISUCasingLights_TrafficLightRoadSideNL_5/1
  TrafficLightRoadSideNL_5_Casing.LightRed_Control_Mux/1(Bus) -> TrafficLightRoadSideNL_5_Casing.LightRed_Control/1
  TrafficLightRoadSideNL_5_Casing.LightRed_SPDIndex/1 -> TrafficLightRoadSideNL_5_Casing.LightRed_Control_Mux/1(SPDIndex [-])
  TrafficLightRoadSideNL_5_Casing.LightRed_Power/1 -> TrafficLightRoadSideNL_5_Casing.LightRed_Control_Mux/2(Power [W])
  TrafficLightRoadSideNL_5_Casing.LightOrange_Control_Mux/1(Bus) -> TrafficLightRoadSideNL_5_Casing.LightOrange_Control/1
  TrafficLightRoadSideNL_5_Casing.LightOrange_SPDIndex/1 -> TrafficLightRoadSideNL_5_Casing.LightOrange_Control_Mux/1(SPDIndex [-])
  TrafficLightRoadSideNL_5_Casing.LightOrange_Power/1 -> TrafficLightRoadSideNL_5_Casing.LightOrange_Control_Mux/2(Power [W])
  TrafficLightRoadSideNL_5_Casing.LightGreen_Control_Mux/1(Bus) -> TrafficLightRoadSideNL_5_Casing.LightGreen_Control/1
  TrafficLightRoadSideNL_5_Casing.LightGreen_SPDIndex/1 -> TrafficLightRoadSideNL_5_Casing.LightGreen_Control_Mux/1(SPDIndex [-])
  TrafficLightRoadSideNL_5_Casing.LightGreen_Power/1 -> TrafficLightRoadSideNL_5_Casing.LightGreen_Control_Mux/2(Power [W])
  Ground_1/1 -> VISUCasingLights_Mux/1(Green [-])
  Ground_2/1 -> VISUCasingLights_Mux/2(Orange [-])
  Ground_3/1 -> VISUCasingLights_Mux/3(Red [-])

== system W02_Base_Map_PB_cs/TrafficLightRoadSideNL_5_Casing.LightGreen_Control ==
  TrafficLightRoadSideNL_5_Casing.LightGreen_Control : Inport  Tag=inport/plugin/sfun_PBCLight  OutDataTypeStr=Bus: PRESCAN_PBCLIGHT_DATA  PortDimensions=1  SampleTime=0.05  BusOutputAsStruct=on
  Actuator : S-Function  LoadFcn=addpath 'C:/Program Files/Simcenter Prescan/Prescan_2019.2/Plugins/PBCameraPlugin/matlab';addpath 'C:/Program Files/Simcenter Prescan/Prescan_2019.2/Plugins/PBCameraPlugin/bin';load('PreScanPBCLightData.mat');  FunctionName=sfun_PBCLight  Parameters=lightID, timestepMask  SFunctionDeploymentMode=off  EnableBusSupport=off  mask(Physics Based Camera plugin block){lightID=14, timestepMask=0.05}
      mask prompts: lightID "Light ID:"; timestepMask "MATLAB timestep:"
      mask help: Light Control I/O
      mask Help: eval('openHelp(6500)')
      mask Display: image(imread('ico_PBCControl.png'))
  wires:
  TrafficLightRoadSideNL_5_Casing.LightGreen_Control/1 -> Actuator/1

== system W02_Base_Map_PB_cs/TrafficLightRoadSideNL_5_Casing.LightOrange_Control ==
  TrafficLightRoadSideNL_5_Casing.LightOrange_Control : Inport  Tag=inport/plugin/sfun_PBCLight  OutDataTypeStr=Bus: PRESCAN_PBCLIGHT_DATA  PortDimensions=1  SampleTime=0.05  BusOutputAsStruct=on
  Actuator : S-Function  LoadFcn=addpath 'C:/Program Files/Simcenter Prescan/Prescan_2019.2/Plugins/PBCameraPlugin/matlab';addpath 'C:/Program Files/Simcenter Prescan/Prescan_2019.2/Plugins/PBCameraPlugin/bin';load('PreScanPBCLightData.mat');  FunctionName=sfun_PBCLight  Parameters=lightID, timestepMask  SFunctionDeploymentMode=off  EnableBusSupport=off  mask(Physics Based Camera plugin block){lightID=13, timestepMask=0.05}
      mask prompts: lightID "Light ID:"; timestepMask "MATLAB timestep:"
      mask help: Light Control I/O
      mask Help: eval('openHelp(6500)')
      mask Display: image(imread('ico_PBCControl.png'))
  wires:
  TrafficLightRoadSideNL_5_Casing.LightOrange_Control/1 -> Actuator/1

== system W02_Base_Map_PB_cs/TrafficLightRoadSideNL_5_Casing.LightRed_Control ==
  TrafficLightRoadSideNL_5_Casing.LightRed_Control : Inport  Tag=inport/plugin/sfun_PBCLight  OutDataTypeStr=Bus: PRESCAN_PBCLIGHT_DATA  PortDimensions=1  SampleTime=0.05  BusOutputAsStruct=on
  Actuator : S-Function  LoadFcn=addpath 'C:/Program Files/Simcenter Prescan/Prescan_2019.2/Plugins/PBCameraPlugin/matlab';addpath 'C:/Program Files/Simcenter Prescan/Prescan_2019.2/Plugins/PBCameraPlugin/bin';load('PreScanPBCLightData.mat');  FunctionName=sfun_PBCLight  Parameters=lightID, timestepMask  SFunctionDeploymentMode=off  EnableBusSupport=off  mask(Physics Based Camera plugin block){lightID=12, timestepMask=0.05}
      mask prompts: lightID "Light ID:"; timestepMask "MATLAB timestep:"
      mask help: Light Control I/O
      mask Help: eval('openHelp(6500)')
      mask Display: image(imread('ico_PBCControl.png'))
  wires:
  TrafficLightRoadSideNL_5_Casing.LightRed_Control/1 -> Actuator/1

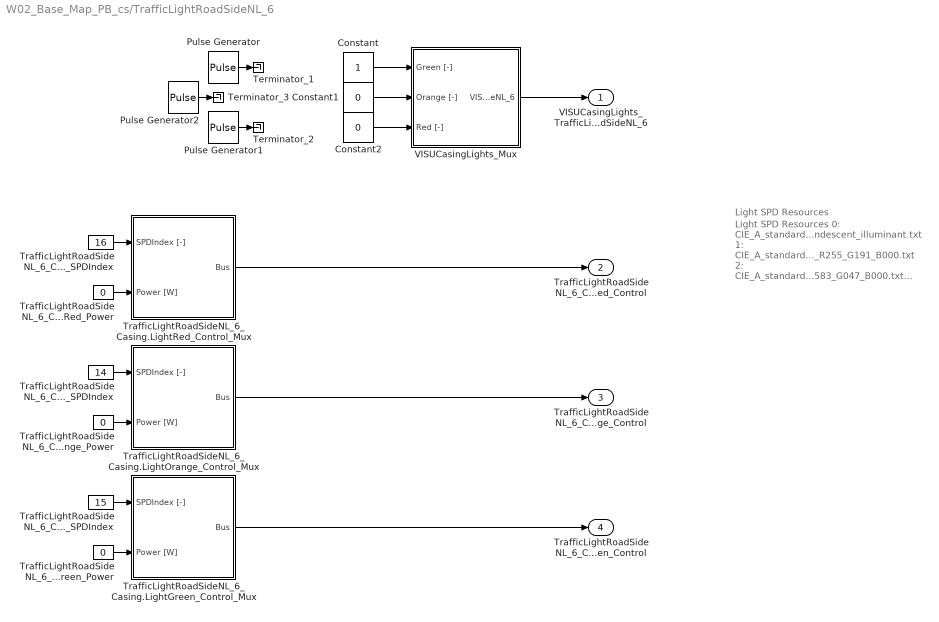
== system W02_Base_Map_PB_cs/TrafficLightRoadSideNL_6 ==
  note: Light SPD Resources
      |
      |  0: CIE_A_standard_incandescent_illuminant.txt
      |  1: CIE_A_standard_incandescent_illuminant.txt_x_R255_G191_B000.txt
      |  2: CIE_A_standard_incandescent_illuminant.txt_x_R583_G047_B000.txt
      |  3: CIE_F12_standard_fluorescent_illuminant.txt
      |  4: Illuminant_D65.txt
      |  5: Light_SPD_H1_12_8V_Filament.txt
      |  6: Light_SPD_H1_13_2V_Filament.txt
      |  7: Light_SPD_H11_12V_Filament.txt
      |  8: Light_SPD_H7_12_8V_Filament.txt
      |  9: Light_SPD_H7_13_2V_Filament.txt
      | 10: Light_SPD_H8_13_2V_Filament.txt
      | 11: Light_SPD_Halogen.txt
      | 12: Light_SPD_High_Power_LED.txt
      | 13: Light_SPD_HPS_High_Pressure_Sodium.txt
      | 14: Light_SPD_incandescent_traffic_signal_amber.txt
      | 15: Light_SPD_incandescent_traffic_signal_green.txt
      | 16: Light_SPD_incandescent_traffic_signal_red.txt
      | 17: Light_SPD_LED_D1S_HID.txt
      | 18: Light_SPD_LED_traffic_signal_amber.txt
      | 19: Light_SPD_LED_traffic_signal_green.txt
      | 20: Light_SPD_LED_traffic_signal_red.txt
      | 21: Light_SPD_LPS_Low_Pressure_Sodium.txt
      | 22: Light_SPD_Mercury.txt
      | 23: Light_SPD_Reddish_Neon_Sign.txt
      | 24: Noma_Twister_Blue_13W_120V.txt
      | 25: Philips_Blue_Golite_P1_Apollo_1750Lux.txt
      | 26: SPD_flat_1.0.txt
  note: Light SPD Resources
  Constant : Constant
  Constant1 : Constant  Value=0
  Constant2 : Constant  Value=0
  Pulse Generator : DiscretePulseGenerator  PulseType=Time based  Period=10  PulseWidth=40
  Pulse Generator1 : DiscretePulseGenerator  PulseType=Time based  Period=10  PulseWidth=40  PhaseDelay=6
  Pulse Generator2 : DiscretePulseGenerator  PulseType=Time based  Period=10  PulseWidth=20  PhaseDelay=4
  Terminator_1 : Terminator
  Terminator_2 : Terminator
  Terminator_3 : Terminator
  TrafficLightRoadSideNL_6_Casing.LightGreen_Control_Mux : Subsystem  Tag=mux/plugin/LightSignals
  TrafficLightRoadSideNL_6_Casing.LightGreen_Power : Constant  Tag=TrafficLightRoadSideNL_6_Casing.LightGreen_Power  Value=0
  TrafficLightRoadSideNL_6_Casing.LightGreen_SPDIndex : Constant  Tag=TrafficLightRoadSideNL_6_Casing.LightGreen_SPDIndex  Value=15
  TrafficLightRoadSideNL_6_Casing.LightOrange_Control_Mux : Subsystem  Tag=mux/plugin/LightSignals
  TrafficLightRoadSideNL_6_Casing.LightOrange_Power : Constant  Tag=TrafficLightRoadSideNL_6_Casing.LightOrange_Power  Value=0
  TrafficLightRoadSideNL_6_Casing.LightOrange_SPDIndex : Constant  Tag=TrafficLightRoadSideNL_6_Casing.LightOrange_SPDIndex  Value=14
  TrafficLightRoadSideNL_6_Casing.LightRed_Control_Mux : Subsystem  Tag=mux/plugin/LightSignals
  TrafficLightRoadSideNL_6_Casing.LightRed_Power : Constant  Tag=TrafficLightRoadSideNL_6_Casing.LightRed_Power  Value=0
  TrafficLightRoadSideNL_6_Casing.LightRed_SPDIndex : Constant  Tag=TrafficLightRoadSideNL_6_Casing.LightRed_SPDIndex  Value=16
  VISUCasingLights_Mux : Subsystem  Tag=mux/VisuCasingLights  mask(PreScan User Interface: VisuTrafficLight){}
      mask help:
      | The VisuTrafficLight block provides a way to animate traffic lights: switch on and off individual lights.
      |
      | For more information, please click Help.
      mask Help: eval('openHelp(731)')
  VISUCasingLights_TrafficLightRoadSideNL_6 : Outport  Tag=outport/VisuCasingLights  SampleTime=1/300
  TrafficLightRoadSideNL_6_Casing.LightRed_Control : Outport  Tag=outport/plugin/sfun_PBCLight  Port=2  OutDataTypeStr=Bus: PRESCAN_PBCLIGHT_DATA  PortDimensions=1  SampleTime=0.05
  TrafficLightRoadSideNL_6_Casing.LightOrange_Control : Outport  Tag=outport/plugin/sfun_PBCLight  Port=3  OutDataTypeStr=Bus: PRESCAN_PBCLIGHT_DATA  PortDimensions=1  SampleTime=0.05
  TrafficLightRoadSideNL_6_Casing.LightGreen_Control : Outport  Tag=outport/plugin/sfun_PBCLight  Port=4  OutDataTypeStr=Bus: PRESCAN_PBCLIGHT_DATA  PortDimensions=1  SampleTime=0.05
  wires:
  Constant/1 -> VISUCasingLights_Mux/1(Green [-])
  Constant1/1 -> VISUCasingLights_Mux/2(Orange [-])
  Constant2/1 -> VISUCasingLights_Mux/3(Red [-])
  VISUCasingLights_Mux/1(VISUCasingLights_TrafficLightRoadSideNL_6) -> VISUCasingLights_TrafficLightRoadSideNL_6/1
  TrafficLightRoadSideNL_6_Casing.LightRed_Control_Mux/1(Bus) -> TrafficLightRoadSideNL_6_Casing.LightRed_Control/1
  TrafficLightRoadSideNL_6_Casing.LightRed_SPDIndex/1 -> TrafficLightRoadSideNL_6_Casing.LightRed_Control_Mux/1(SPDIndex [-])
  TrafficLightRoadSideNL_6_Casing.LightRed_Power/1 -> TrafficLightRoadSideNL_6_Casing.LightRed_Control_Mux/2(Power [W])
  TrafficLightRoadSideNL_6_Casing.LightOrange_Control_Mux/1(Bus) -> TrafficLightRoadSideNL_6_Casing.LightOrange_Control/1
  TrafficLightRoadSideNL_6_Casing.LightOrange_SPDIndex/1 -> TrafficLightRoadSideNL_6_Casing.LightOrange_Control_Mux/1(SPDIndex [-])
  TrafficLightRoadSideNL_6_Casing.LightOrange_Power/1 -> TrafficLightRoadSideNL_6_Casing.LightOrange_Control_Mux/2(Power [W])
  TrafficLightRoadSideNL_6_Casing.LightGreen_Control_Mux/1(Bus) -> TrafficLightRoadSideNL_6_Casing.LightGreen_Control/1
  TrafficLightRoadSideNL_6_Casing.LightGreen_SPDIndex/1 -> TrafficLightRoadSideNL_6_Casing.LightGreen_Control_Mux/1(SPDIndex [-])
  TrafficLightRoadSideNL_6_Casing.LightGreen_Power/1 -> TrafficLightRoadSideNL_6_Casing.LightGreen_Control_Mux/2(Power [W])
  Pulse Generator/1 -> Terminator_1/1
  Pulse Generator1/1 -> Terminator_2/1
  Pulse Generator2/1 -> Terminator_3/1

== system W02_Base_Map_PB_cs/TrafficLightRoadSideNL_6_Casing.LightGreen_Control ==
  TrafficLightRoadSideNL_6_Casing.LightGreen_Control : Inport  Tag=inport/plugin/sfun_PBCLight  OutDataTypeStr=Bus: PRESCAN_PBCLIGHT_DATA  PortDimensions=1  SampleTime=0.05  BusOutputAsStruct=on
  Actuator : S-Function  LoadFcn=addpath 'C:/Program Files/Simcenter Prescan/Prescan_2019.2/Plugins/PBCameraPlugin/matlab';addpath 'C:/Program Files/Simcenter Prescan/Prescan_2019.2/Plugins/PBCameraPlugin/bin';load('PreScanPBCLightData.mat');  FunctionName=sfun_PBCLight  Parameters=lightID, timestepMask  SFunctionDeploymentMode=off  EnableBusSupport=off  mask(Physics Based Camera plugin block){lightID=23, timestepMask=0.05}
      mask prompts: lightID "Light ID:"; timestepMask "MATLAB timestep:"
      mask help: Light Control I/O
      mask Help: eval('openHelp(6500)')
      mask Display: image(imread('ico_PBCControl.png'))
  wires:
  TrafficLightRoadSideNL_6_Casing.LightGreen_Control/1 -> Actuator/1

== system W02_Base_Map_PB_cs/TrafficLightRoadSideNL_6_Casing.LightOrange_Control ==
  TrafficLightRoadSideNL_6_Casing.LightOrange_Control : Inport  Tag=inport/plugin/sfun_PBCLight  OutDataTypeStr=Bus: PRESCAN_PBCLIGHT_DATA  PortDimensions=1  SampleTime=0.05  BusOutputAsStruct=on
  Actuator : S-Function  LoadFcn=addpath 'C:/Program Files/Simcenter Prescan/Prescan_2019.2/Plugins/PBCameraPlugin/matlab';addpath 'C:/Program Files/Simcenter Prescan/Prescan_2019.2/Plugins/PBCameraPlugin/bin';load('PreScanPBCLightData.mat');  FunctionName=sfun_PBCLight  Parameters=lightID, timestepMask  SFunctionDeploymentMode=off  EnableBusSupport=off  mask(Physics Based Camera plugin block){lightID=22, timestepMask=0.05}
      mask prompts: lightID "Light ID:"; timestepMask "MATLAB timestep:"
      mask help: Light Control I/O
      mask Help: eval('openHelp(6500)')
      mask Display: image(imread('ico_PBCControl.png'))
  wires:
  TrafficLightRoadSideNL_6_Casing.LightOrange_Control/1 -> Actuator/1

== system W02_Base_Map_PB_cs/TrafficLightRoadSideNL_6_Casing.LightRed_Control ==
  TrafficLightRoadSideNL_6_Casing.LightRed_Control : Inport  Tag=inport/plugin/sfun_PBCLight  OutDataTypeStr=Bus: PRESCAN_PBCLIGHT_DATA  PortDimensions=1  SampleTime=0.05  BusOutputAsStruct=on
  Actuator : S-Function  LoadFcn=addpath 'C:/Program Files/Simcenter Prescan/Prescan_2019.2/Plugins/PBCameraPlugin/matlab';addpath 'C:/Program Files/Simcenter Prescan/Prescan_2019.2/Plugins/PBCameraPlugin/bin';load('PreScanPBCLightData.mat');  FunctionName=sfun_PBCLight  Parameters=lightID, timestepMask  SFunctionDeploymentMode=off  EnableBusSupport=off  mask(Physics Based Camera plugin block){lightID=21, timestepMask=0.05}
      mask prompts: lightID "Light ID:"; timestepMask "MATLAB timestep:"
      mask help: Light Control I/O
      mask Help: eval('openHelp(6500)')
      mask Display: image(imread('ico_PBCControl.png'))
  wires:
  TrafficLightRoadSideNL_6_Casing.LightRed_Control/1 -> Actuator/1
